simulink model "Standing_Strategy"  (R2025a)
settings: Solver=ode23t  StartTime=0.0  StopTime=4.0  MaxStep=0.01  RelTol=1e-3
InitFcn:
  | params;
values from neighbouring files (symbols this model uses):
  ankle = []    [params.m]
  arm = []    [params.m]
  F_inp = 70    [params.m]
  foot = []    [params.m]
  g = 9.81    [params.m]
  heel = []    [params.m]
  hip_joint = []    [params.m]
  leg = []    [params.m]
  mp = []    [params.m]
  shoulder = []    [params.m]
  sol = []    [params.m]
  ta = []    [params.m]
  torso = []    [params.m]
undefined symbols (not defined in the file or in its folder): X, Y, Z
libraries: sm_lib x43, nesl_utility x13, dlactivationlib x2
(part 2 of 2)

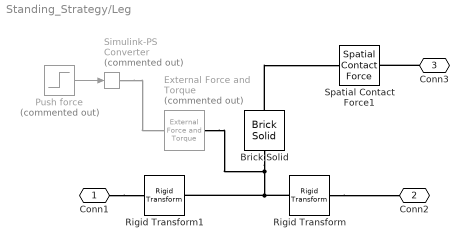
== system Standing_Strategy/Leg ==
  Brick Solid : sm_lib/Body Elements/Brick Solid  BrickDimensions=[L W H]  BrickDimensionsUnits=m  ExportEntireGeometry=on  InertiaType=CalculateFromGeometry  BasedOnType=Density  Density=rho  DensityUnits=g/cm^3  Mass=1  MassUnits=kg  CenterOfMass=[0 0 0]  CenterOfMassUnits=m  MomentsOfInertia=[1 1 1]  MomentsOfInertiaUnits=kg*m^2  ProductsOfInertia=[0 0 0]  ProductsOfInertiaUnits=kg*m^2  GraphicType=FromGeometry  MarkerShape=Sphere  MarkerSize=10  GraphicVisPropType=SimpleVisualProperties  GraphicDiffuseColor=rgb  GraphicOpacity=1  GraphicSpecularColor=[0.5 0.5 0.5 1.0]  GraphicAmbientColor=[0.15 0.15 0.15 1.0]  GraphicEmissiveColor=[0.0 0.0 0.0 1.0]  GraphicShininess=75  DoExposeReferenceFrame=on  SerializedFrames=<Frames/>
  External Force and Torque : sm_lib/Forces and Torques/External Force and Torque  Commented=on  EnableForceX=off  EnableForceY=off  EnableForceZ=on  EnableForce=off  ForceResolutionFrame=AttachedFrame  EnableTorqueX=off  EnableTorqueY=off  EnableTorqueZ=off  EnableTorque=off  TorqueResolutionFrame=AttachedFrame
  Push force : Step  Commented=on  Time=0.1  Before=-300  After=0  SampleTime=0
  Rigid Transform : sm_lib/Frames and Transforms/Rigid Transform  RotationMethod=None  FollAlignAxisA=+X  BaseAlignAxisA=+Y  FollAlignAxisB=+Y  BaseAlignAxisB=+Z  RotationStandardAxis=+Y  RotationAngle=-90  RotationAngleUnits=deg  RotationArbitraryAxis=[0 0 1]  RotationSequenceAxes=FollowerAxes  RotationSequence=XYX  RotationSequenceAngles=[0 0 0]  RotationSequenceAnglesUnits=deg  RotationMatrix=[1 0 0; 0 1 0; 0 0 1]  Quaternion=[1 0 0 0]  TranslationMethod=StandardAxis  TranslationCartesianOffset=[0 0 0]  TranslationCartesianOffsetUnits=m  TranslationStandardAxis=+X  TranslationStandardOffset=L/2  TranslationStandardOffsetUnits=m  TranslationROffset=0  TranslationROffsetUnits=m  TranslationThetaOffset=0  TranslationThetaOffsetUnits=deg  TranslationZOffset=0  TranslationZOffsetUnits=m
  Rigid Transform1 : sm_lib/Frames and Transforms/Rigid Transform  RotationMethod=None  FollAlignAxisA=+X  BaseAlignAxisA=+Y  FollAlignAxisB=+Y  BaseAlignAxisB=+Z  RotationStandardAxis=+Y  RotationAngle=-90  RotationAngleUnits=deg  RotationArbitraryAxis=[0 0 1]  RotationSequenceAxes=FollowerAxes  RotationSequence=XYX  RotationSequenceAngles=[0 0 0]  RotationSequenceAnglesUnits=deg  RotationMatrix=[1 0 0; 0 1 0; 0 0 1]  Quaternion=[1 0 0 0]  TranslationMethod=StandardAxis  TranslationCartesianOffset=[0 0 0]  TranslationCartesianOffsetUnits=m  TranslationStandardAxis=-X  TranslationStandardOffset=L/2  TranslationStandardOffsetUnits=m  TranslationROffset=0  TranslationROffsetUnits=m  TranslationThetaOffset=0  TranslationThetaOffsetUnits=deg  TranslationZOffset=0  TranslationZOffsetUnits=m
  Simulink-PS Converter : nesl_utility/Simulink-PS Converter  Commented=on  PhysicalDomain=network_engine_domain  SubClassName=ps_input  LeftPortType=input  RightPortType=output  PseudoPeriodic=off  Frequencies=[]  NoiseDistribution=none  NoiseParameters=[]  Unit=1  AffineConversion=off  FilteringAndDerivatives=provide  SimscapeFilterOrder=1  InputFilterTimeConstant=0.001  UdotUserProvided=0
  Spatial Contact Force1 : sm_lib/Forces and Torques/Spatial Contact Force  SenseSeparationDistance=off  NormalForceType=SmoothSpringDamper  NormalStiffness=1e6  NormalStiffnessUnits=N/m  NormalDamping=1e3  NormalDampingUnits=N/(m/s)  NormalTransitionRegionWidth=1e-4  NormalTransitionRegionWidthUnits=m  FrictionType=SmoothStickSlip  CoefficientOfStaticFriction=0.2  CoefficientOfDynamicFriction=0.1  FrictionalCriticalVelocity=1e-3  FrictionalCriticalVelocityUnits=m/s  SenseContactSignal=off  SensePenetrationDepth=off  SenseNormalVelocity=off  SenseTangentialVelocity=off  SensingForceTorqueDirection=BaseOnFollower  SensingForceTorqueResolutionFrame=ContactFrame  SenseNormalForce=off  SenseNormalForceMagnitude=off  SenseNormalTorque=off  SenseFrictionalForce=off  SenseFrictionalForceMagnitude=off  SenseFrictionalTorque=off  SenseTotalForce=off  SenseTotalTorque=off  SenseContactBaseRotation=off  SenseContactBaseTranslation=off  SenseContactFollowerRotation=off  SenseContactFollowerTranslation=off  ZeroCrossDetectContactStartAndEnd=off
  Conn1 : PMIOPort  Side=Left
  Conn2 : PMIOPort  Port=2  Side=Right
  Conn3 : PMIOPort  Port=3  Side=Right
  wires:
  Push force/1 -> Simulink-PS Converter/1
  connections:
  Rigid Transform/RConn1 -- Conn2/RConn1
  Conn1/RConn1 -- Rigid Transform1/RConn1
  Brick Solid/RConn1 -- External Force and Torque/RConn1 -- Rigid Transform/LConn1 -- Rigid Transform1/LConn1
  Brick Solid/LConn1 -- Spatial Contact Force1/RConn1
  Conn3/RConn1 -- Spatial Contact Force1/LConn1
  Simulink-PS Converter/RConn1 -- External Force and Torque/LConn1

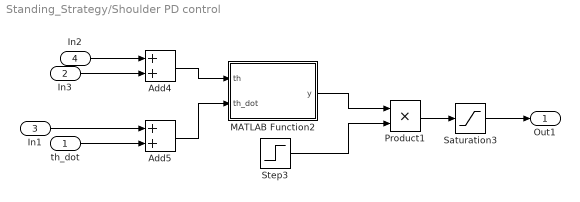
== system Standing_Strategy/Shoulder PD control ==
  th_dot : Inport
  In3 : Inport  Port=2
  In1 : Inport  Port=3
  In2 : Inport  Port=4
  Add4 : Sum
  Add5 : Sum
  MATLAB Function2 : MATLAB Function  TreatAsAtomicUnit=on
  Product1 : Product
  Saturation3 : Saturate  UpperLimit=50  LowerLimit=-50
  Step3 : Step  Time=10*hip_joint.T2  SampleTime=0
  Out1 : Outport
  wires:
  Product1/1 -> Saturation3/1
  Add5/1 -> MATLAB Function2/2(th_dot)
  In1/1 -> Add5/1
  Step3/1 -> Product1/2
  Add4/1 -> MATLAB Function2/1(th)
  In2/1 -> Add4/1
  MATLAB Function2/1(y) -> Product1/1
  In3/1 -> Add4/2
  th_dot/1 -> Add5/2
  Saturation3/1 -> Out1/1

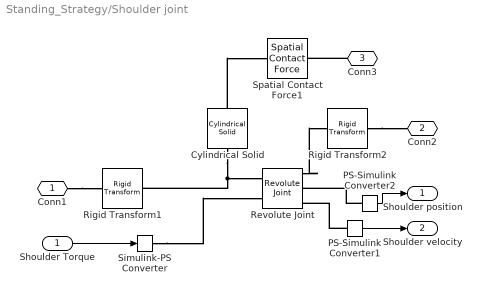
== system Standing_Strategy/Shoulder joint ==
  Shoulder Torque : Inport
  Cylindrical Solid : sm_lib/Body Elements/Cylindrical Solid  CylinderRadius=R  CylinderRadiusUnits=m  CylinderLength=L  CylinderLengthUnits=m  ExportEntireGeometry=on  InertiaType=CalculateFromGeometry  BasedOnType=Density  Density=rho  DensityUnits=g/cm^3  Mass=1  MassUnits=kg  CenterOfMass=[0 0 0]  CenterOfMassUnits=m  MomentsOfInertia=[1 1 1]  MomentsOfInertiaUnits=kg*m^2  ProductsOfInertia=[0 0 0]  ProductsOfInertiaUnits=kg*m^2  GraphicType=FromGeometry  MarkerShape=Sphere  MarkerSize=10  GraphicVisPropType=SimpleVisualProperties  GraphicDiffuseColor=rgb  GraphicOpacity=1  GraphicSpecularColor=[0.5 0.5 0.5 1.0]  GraphicAmbientColor=[0.15 0.15 0.15 1.0]  GraphicEmissiveColor=[0.0 0.0 0.0 1.0]  GraphicShininess=75  DoExposeReferenceFrame=on  SerializedFrames=<Frames/>
  PS-Simulink Converter1 : nesl_utility/PS-Simulink Converter  PhysicalDomain=network_engine_domain  SubClassName=ps_output  LeftPortType=input  RightPortType=output  PseudoPeriodic=off  Frequencies=[]  VectorFormat=inherit  Unit=inherit  AffineConversion=off
  PS-Simulink Converter2 : nesl_utility/PS-Simulink Converter  PhysicalDomain=network_engine_domain  SubClassName=ps_output  LeftPortType=input  RightPortType=output  PseudoPeriodic=off  Frequencies=[]  VectorFormat=inherit  Unit=inherit  AffineConversion=off
  Revolute Joint : sm_lib/Joints/Revolute Joint  JointMode=Normal  CompositeWrenchDir=FollowerOnBase  CompositeWrenchFrame=BaseFrame  SenseConstraintForce=off  SenseConstraintTorque=off  SenseTotalForce=off  SenseTotalTorque=off  PositionTargetSpecify=on  PositionTargetPriority=High  PositionTargetValue=shoulder.th_init  PositionTargetValueUnits=rad  VelocityTargetSpecify=off  VelocityTargetPriority=High  VelocityTargetValue=0  VelocityTargetValueUnits=deg/s  EquilibriumPosition=shoulder.th_init  EquilibriumPositionUnits=rad  SpringStiffness=0  SpringStiffnessUnits=N*m/deg  DampingCoefficient=0.1  DampingCoefficientUnits=N*m/(deg/s)  LowerLimitSpecify=off  LowerLimitBound=0  LowerLimitBoundUnits=deg  LowerLimitStiffness=1e4  LowerLimitStiffnessUnits=N*m/deg  LowerLimitDamping=10  LowerLimitDampingUnits=N*m/(deg/s)  LowerLimitTransitionRegionWidth=0.1  LowerLimitTransitionRegionWidthUnits=deg  UpperLimitSpecify=off  UpperLimitBound=120  UpperLimitBoundUnits=deg  UpperLimitStiffness=1e4  UpperLimitStiffnessUnits=N*m/deg  UpperLimitDamping=10  UpperLimitDampingUnits=N*m/(deg/s)  UpperLimitTransitionRegionWidth=0.1  UpperLimitTransitionRegionWidthUnits=deg  TorqueActuationMode=InputTorque  MotionActuationMode=ComputedMotion  SensePosition=on  SenseVelocity=on  SenseAcceleration=off  SenseTorqueForce=off  SenseLowerLimitTorqueForce=off  SenseUpperLimitTorqueForce=off
  Rigid Transform1 : sm_lib/Frames and Transforms/Rigid Transform  RotationMethod=StandardAxis  FollAlignAxisA=+X  BaseAlignAxisA=+Y  FollAlignAxisB=+Y  BaseAlignAxisB=+Z  RotationStandardAxis=+X  RotationAngle=90  RotationAngleUnits=deg  RotationArbitraryAxis=[0 0 1]  RotationSequenceAxes=FollowerAxes  RotationSequence=XYX  RotationSequenceAngles=[0 0 0]  RotationSequenceAnglesUnits=deg  RotationMatrix=[1 0 0; 0 1 0; 0 0 1]  Quaternion=[1 0 0 0]  TranslationMethod=StandardAxis  TranslationCartesianOffset=[0 0 0]  TranslationCartesianOffsetUnits=m  TranslationStandardAxis=-X  TranslationStandardOffset=R  TranslationStandardOffsetUnits=m  TranslationROffset=0  TranslationROffsetUnits=m  TranslationThetaOffset=0  TranslationThetaOffsetUnits=deg  TranslationZOffset=0  TranslationZOffsetUnits=m
  Rigid Transform2 : sm_lib/Frames and Transforms/Rigid Transform  RotationMethod=StandardAxis  FollAlignAxisA=+X  BaseAlignAxisA=+Y  FollAlignAxisB=+Y  BaseAlignAxisB=+Z  RotationStandardAxis=-X  RotationAngle=90  RotationAngleUnits=deg  RotationArbitraryAxis=[0 0 1]  RotationSequenceAxes=FollowerAxes  RotationSequence=XYX  RotationSequenceAngles=[0 0 0]  RotationSequenceAnglesUnits=deg  RotationMatrix=[1 0 0; 0 1 0; 0 0 1]  Quaternion=[1 0 0 0]  TranslationMethod=StandardAxis  TranslationCartesianOffset=[0 0 0]  TranslationCartesianOffsetUnits=m  TranslationStandardAxis=-X  TranslationStandardOffset=R  TranslationStandardOffsetUnits=m  TranslationROffset=0  TranslationROffsetUnits=m  TranslationThetaOffset=0  TranslationThetaOffsetUnits=deg  TranslationZOffset=0  TranslationZOffsetUnits=m
  Simulink-PS Converter : nesl_utility/Simulink-PS Converter  PhysicalDomain=network_engine_domain  SubClassName=ps_input  LeftPortType=input  RightPortType=output  PseudoPeriodic=off  Frequencies=[]  NoiseDistribution=none  NoiseParameters=[]  Unit=1  AffineConversion=off  FilteringAndDerivatives=provide  SimscapeFilterOrder=1  InputFilterTimeConstant=0.001  UdotUserProvided=0
  Spatial Contact Force1 : sm_lib/Forces and Torques/Spatial Contact Force  SenseSeparationDistance=off  NormalForceType=SmoothSpringDamper  NormalStiffness=1e6  NormalStiffnessUnits=N/m  NormalDamping=1e3  NormalDampingUnits=N/(m/s)  NormalTransitionRegionWidth=1e-4  NormalTransitionRegionWidthUnits=m  FrictionType=SmoothStickSlip  CoefficientOfStaticFriction=0.2  CoefficientOfDynamicFriction=0.1  FrictionalCriticalVelocity=1e-3  FrictionalCriticalVelocityUnits=m/s  SenseContactSignal=off  SensePenetrationDepth=off  SenseNormalVelocity=off  SenseTangentialVelocity=off  SensingForceTorqueDirection=BaseOnFollower  SensingForceTorqueResolutionFrame=ContactFrame  SenseNormalForce=off  SenseNormalForceMagnitude=off  SenseNormalTorque=off  SenseFrictionalForce=off  SenseFrictionalForceMagnitude=off  SenseFrictionalTorque=off  SenseTotalForce=off  SenseTotalTorque=off  SenseContactBaseRotation=off  SenseContactBaseTranslation=off  SenseContactFollowerRotation=off  SenseContactFollowerTranslation=off  ZeroCrossDetectContactStartAndEnd=off
  Conn1 : PMIOPort  Side=Left
  Conn2 : PMIOPort  Port=2  Side=Right
  Conn3 : PMIOPort  Port=3  Side=Right
  Shoulder position : Outport
  Shoulder velocity : Outport  Port=2
  wires:
  PS-Simulink Converter1/1 -> Shoulder velocity/1
  Shoulder Torque/1 -> Simulink-PS Converter/1
  PS-Simulink Converter2/1 -> Shoulder position/1
  connections:
  Conn1/RConn1 -- Rigid Transform1/RConn1
  Cylindrical Solid/RConn1 -- Rigid Transform1/LConn1 -- Revolute Joint/LConn1
  Cylindrical Solid/LConn1 -- Spatial Contact Force1/RConn1
  Conn3/RConn1 -- Spatial Contact Force1/LConn1
  Rigid Transform2/LConn1 -- Conn2/RConn1
  Revolute Joint/RConn1 -- Rigid Transform2/RConn1
  PS-Simulink Converter1/LConn1 -- Revolute Joint/RConn3
  Simulink-PS Converter/RConn1 -- Revolute Joint/LConn2
  PS-Simulink Converter2/LConn1 -- Revolute Joint/RConn2

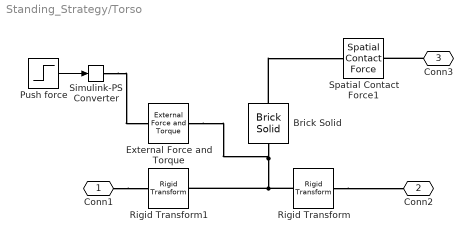
== system Standing_Strategy/Torso ==
  Brick Solid : sm_lib/Body Elements/Brick Solid  BrickDimensions=[L W H]  BrickDimensionsUnits=m  ExportEntireGeometry=on  InertiaType=CalculateFromGeometry  BasedOnType=Density  Density=rho  DensityUnits=g/cm^3  Mass=1  MassUnits=kg  CenterOfMass=[0 0 0]  CenterOfMassUnits=m  MomentsOfInertia=[1 1 1]  MomentsOfInertiaUnits=kg*m^2  ProductsOfInertia=[0 0 0]  ProductsOfInertiaUnits=kg*m^2  GraphicType=FromGeometry  MarkerShape=Sphere  MarkerSize=10  GraphicVisPropType=SimpleVisualProperties  GraphicDiffuseColor=rgb  GraphicOpacity=1  GraphicSpecularColor=[0.5 0.5 0.5 1.0]  GraphicAmbientColor=[0.15 0.15 0.15 1.0]  GraphicEmissiveColor=[0.0 0.0 0.0 1.0]  GraphicShininess=75  DoExposeReferenceFrame=on  SerializedFrames=<Frames/>
  External Force and Torque : sm_lib/Forces and Torques/External Force and Torque  EnableForceX=off  EnableForceY=off  EnableForceZ=on  EnableForce=off  ForceResolutionFrame=AttachedFrame  EnableTorqueX=off  EnableTorqueY=off  EnableTorqueZ=off  EnableTorque=off  TorqueResolutionFrame=AttachedFrame
  Push force : Step  Time=0.1  Before=-F_inp  After=0  SampleTime=0
  Rigid Transform : sm_lib/Frames and Transforms/Rigid Transform  RotationMethod=None  FollAlignAxisA=+X  BaseAlignAxisA=+Y  FollAlignAxisB=+Y  BaseAlignAxisB=+Z  RotationStandardAxis=+Y  RotationAngle=-90  RotationAngleUnits=deg  RotationArbitraryAxis=[0 0 1]  RotationSequenceAxes=FollowerAxes  RotationSequence=XYX  RotationSequenceAngles=[0 0 0]  RotationSequenceAnglesUnits=deg  RotationMatrix=[1 0 0; 0 1 0; 0 0 1]  Quaternion=[1 0 0 0]  TranslationMethod=StandardAxis  TranslationCartesianOffset=[0 0 0]  TranslationCartesianOffsetUnits=m  TranslationStandardAxis=+X  TranslationStandardOffset=L/2  TranslationStandardOffsetUnits=m  TranslationROffset=0  TranslationROffsetUnits=m  TranslationThetaOffset=0  TranslationThetaOffsetUnits=deg  TranslationZOffset=0  TranslationZOffsetUnits=m
  Rigid Transform1 : sm_lib/Frames and Transforms/Rigid Transform  RotationMethod=None  FollAlignAxisA=+X  BaseAlignAxisA=+Y  FollAlignAxisB=+Y  BaseAlignAxisB=+Z  RotationStandardAxis=+Y  RotationAngle=-90  RotationAngleUnits=deg  RotationArbitraryAxis=[0 0 1]  RotationSequenceAxes=FollowerAxes  RotationSequence=XYX  RotationSequenceAngles=[0 0 0]  RotationSequenceAnglesUnits=deg  RotationMatrix=[1 0 0; 0 1 0; 0 0 1]  Quaternion=[1 0 0 0]  TranslationMethod=StandardAxis  TranslationCartesianOffset=[0 0 0]  TranslationCartesianOffsetUnits=m  TranslationStandardAxis=-X  TranslationStandardOffset=L/2  TranslationStandardOffsetUnits=m  TranslationROffset=0  TranslationROffsetUnits=m  TranslationThetaOffset=0  TranslationThetaOffsetUnits=deg  TranslationZOffset=0  TranslationZOffsetUnits=m
  Simulink-PS Converter : nesl_utility/Simulink-PS Converter  PhysicalDomain=network_engine_domain  SubClassName=ps_input  LeftPortType=input  RightPortType=output  PseudoPeriodic=off  Frequencies=[]  NoiseDistribution=none  NoiseParameters=[]  Unit=1  AffineConversion=off  FilteringAndDerivatives=provide  SimscapeFilterOrder=1  InputFilterTimeConstant=0.001  UdotUserProvided=0
  Spatial Contact Force1 : sm_lib/Forces and Torques/Spatial Contact Force  SenseSeparationDistance=off  NormalForceType=SmoothSpringDamper  NormalStiffness=1e6  NormalStiffnessUnits=N/m  NormalDamping=1e3  NormalDampingUnits=N/(m/s)  NormalTransitionRegionWidth=1e-4  NormalTransitionRegionWidthUnits=m  FrictionType=SmoothStickSlip  CoefficientOfStaticFriction=0.2  CoefficientOfDynamicFriction=0.1  FrictionalCriticalVelocity=1e-3  FrictionalCriticalVelocityUnits=m/s  SenseContactSignal=off  SensePenetrationDepth=off  SenseNormalVelocity=off  SenseTangentialVelocity=off  SensingForceTorqueDirection=BaseOnFollower  SensingForceTorqueResolutionFrame=ContactFrame  SenseNormalForce=off  SenseNormalForceMagnitude=off  SenseNormalTorque=off  SenseFrictionalForce=off  SenseFrictionalForceMagnitude=off  SenseFrictionalTorque=off  SenseTotalForce=off  SenseTotalTorque=off  SenseContactBaseRotation=off  SenseContactBaseTranslation=off  SenseContactFollowerRotation=off  SenseContactFollowerTranslation=off  ZeroCrossDetectContactStartAndEnd=off
  Conn1 : PMIOPort  Side=Left
  Conn2 : PMIOPort  Port=2  Side=Right
  Conn3 : PMIOPort  Port=3  Side=Right
  wires:
  Push force/1 -> Simulink-PS Converter/1
  connections:
  Rigid Transform/RConn1 -- Conn2/RConn1
  Conn1/RConn1 -- Rigid Transform1/RConn1
  Brick Solid/RConn1 -- Rigid Transform/LConn1 -- Rigid Transform1/LConn1 -- External Force and Torque/RConn1
  Brick Solid/LConn1 -- Spatial Contact Force1/RConn1
  Conn3/RConn1 -- Spatial Contact Force1/LConn1
  Simulink-PS Converter/RConn1 -- External Force and Torque/LConn1

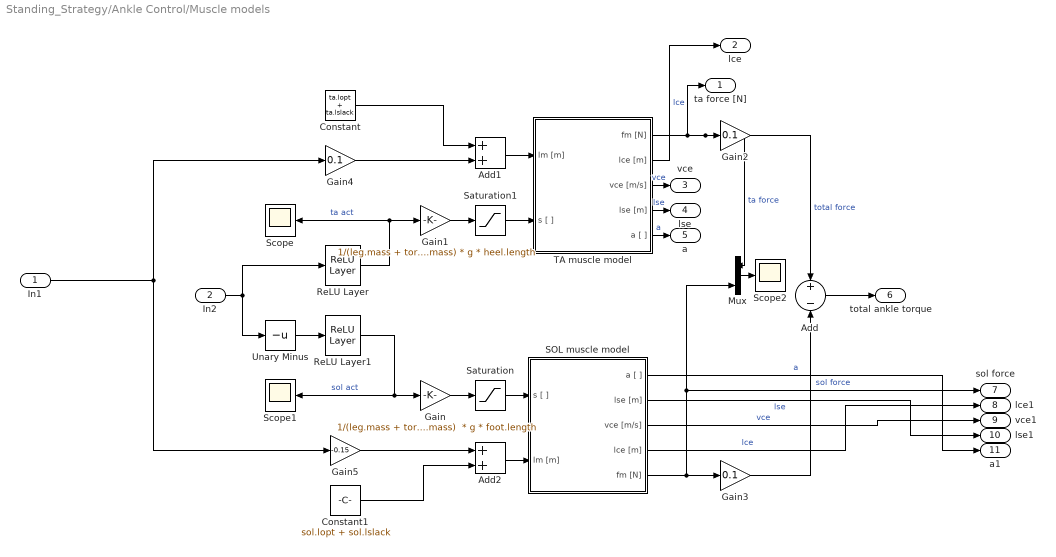
== system Standing_Strategy/Ankle Control/Muscle models ==
  In1 : Inport
  In2 : Inport  Port=2
  Add : Sum  Inputs=+-
  Add1 : Sum
  Add2 : Sum
  Constant : Constant  Value=ta.lopt + ta.lslack
  Constant1 : Constant  Value=sol.lopt + sol.lslack
  Gain : Gain  Gain="1/(leg.mass + torso.mass + arm.mass)  * g * foot.length"
  Gain1 : Gain  Gain=1/(leg.mass + torso.mass + arm.mass) * g * heel.length
  Gain2 : Gain  Gain=0.1
  Gain3 : Gain  Gain=0.1
  Gain4 : Gain  Gain=0.1
  Gain5 : Gain  Gain=-0.15
  Mux : Mux  Inputs=2
  ReLU Layer : dlactivationlib/ReLU Layer  OutMin=[]  OutMax=[]  SampleTime=-1
  ReLU Layer1 : dlactivationlib/ReLU Layer  OutMin=[]  OutMax=[]  SampleTime=-1
  SOL muscle model : Subsystem
  Saturation : Saturate  UpperLimit=1  LowerLimit=0
  Saturation1 : Saturate  UpperLimit=1  LowerLimit=0
  Scope : Scope
      settings: ActiveDisplayYMinimum=-1  ActiveDisplayYMaximum=1  DataLoggingVariableName=ScopeData4
  Scope1 : Scope
      settings: ActiveDisplayYMinimum=-1  ActiveDisplayYMaximum=1  DataLoggingVariableName=ScopeData7
  Scope2 : Scope
      settings: ActiveDisplayYMinimum=-255.71849038678818  ActiveDisplayYMaximum=2301.4664134810942  DataLoggingVariableName=ScopeData8
  TA muscle model : Subsystem
  Unary Minus : UnaryMinus
  ta force [N] : Outport
  lce : Outport  Port=2
  vce : Outport  Port=3
  lse : Outport  Port=4
  a : Outport  Port=5
  total ankle torque : Outport  Port=6
  sol force : Outport  Port=7
  lce1 : Outport  Port=8
  vce1 : Outport  Port=9
  lse1 : Outport  Port=10
  a1 : Outport  Port=11
  wires:
  Mux/1 -> Scope2/1
  Gain3/1 -> Add/2
  Gain2/1 -> Add/1  "total force"
  Add2/1 -> SOL muscle model/2(lm [m])
  TA muscle model/5(a [ ]) -> a/1  "a"
  TA muscle model/1(fm [N]) -> ta force [N]/1, Mux/1, Gain2/1  "ta force"
  Saturation/1 -> SOL muscle model/1(s [ ])
  Constant1/1 -> Add2/2
  Gain5/1 -> Add2/1
  ReLU Layer/1 -> Gain1/1, Scope/1  "ta act"
  SOL muscle model/4(lce [m]) -> lce1/1  "lce"
  In2/1 -> ReLU Layer/1, Unary Minus/1
  SOL muscle model/3(vce [m/s]) -> vce1/1  "vce"
  Add/1 -> total ankle torque/1
  Saturation1/1 -> TA muscle model/2(s [ ])
  Gain1/1 -> Saturation1/1
  SOL muscle model/5(fm [N]) -> sol force/1, Mux/2, Gain3/1  "sol force"
  Gain4/1 -> Add1/2
  ReLU Layer1/1 -> Scope1/1, Gain/1  "sol act"
  In1/1 -> Gain5/1, Gain4/1
  TA muscle model/2(lce [m]) -> lce/1  "lce"
  TA muscle model/4(lse [m]) -> lse/1  "lse"
  SOL muscle model/2(lse [m]) -> lse1/1  "lse"
  Add1/1 -> TA muscle model/1(lm [m])
  TA muscle model/3(vce [m/s]) -> vce/1  "vce"
  Unary Minus/1 -> ReLU Layer1/1
  Constant/1 -> Add1/1
  SOL muscle model/1(a [ ]) -> a1/1  "a"
  Gain/1 -> Saturation/1

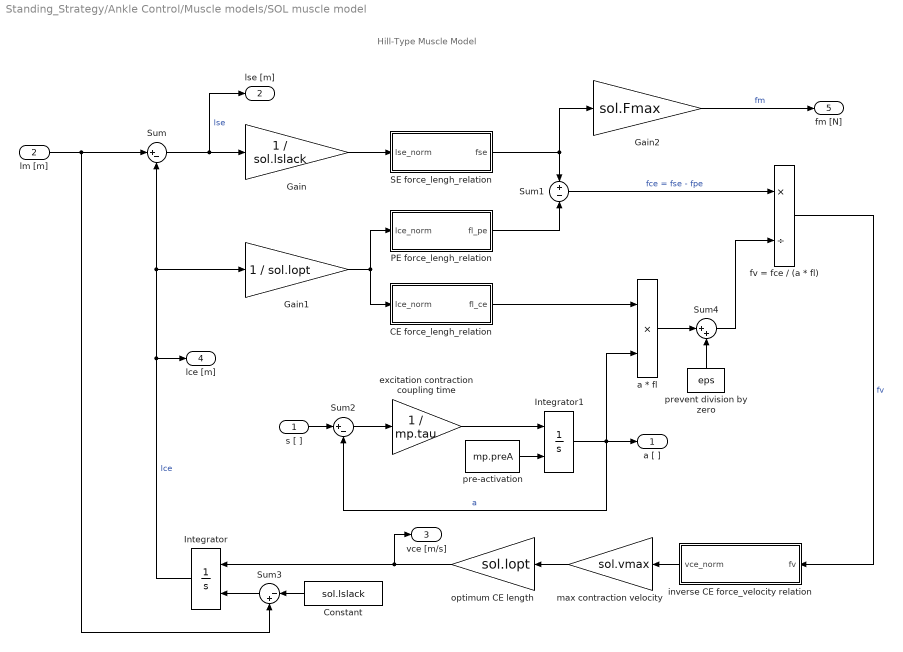
== system Standing_Strategy/Ankle Control/Muscle models/SOL muscle model ==
  note: Hill-Type Muscle Model
  s [ ] : Inport
  lm [m] : Inport  Port=2
  CE force_lengh_relation : MATLAB Function  TreatAsAtomicUnit=on
  Constant : Constant  Value=sol.lslack
  Gain : Gain  Gain=1 / sol.lslack
  Gain1 : Gain  Gain=1 / sol.lopt
  Gain2 : Gain  Gain=sol.Fmax
  Integrator : Integrator  InitialConditionSource=external
  Integrator1 : Integrator  InitialConditionSource=external
  PE force_lengh_relation : MATLAB Function  TreatAsAtomicUnit=on
  SE force_lengh_relation : MATLAB Function  TreatAsAtomicUnit=on
  Sum : Sum  Inputs=|+-
  Sum1 : Sum  Inputs=+-
  Sum2 : Sum  Inputs=|+-
  Sum3 : Sum  Inputs=|-+
  Sum4 : Sum  Inputs=|++
  a * fl : Product  Inputs=**
  excitation contraction coupling time : Gain  Gain=1 / mp.tau
  fv = fce / (a * fl) : Product  Inputs=*/
  inverse CE force_velocity relation : MATLAB Function  TreatAsAtomicUnit=on
  max contraction velocity : Gain  Gain=sol.vmax
  optimum CE length : Gain  Gain=sol.lopt
  pre-activation : Constant  Value=mp.preA
  prevent division by zero : Constant  Value=eps
  a [ ] : Outport
  lse [m] : Outport  Port=2
  vce [m/s] : Outport  Port=3
  lce [m] : Outport  Port=4
  fm [N] : Outport  Port=5
  wires:
  Gain2/1 -> fm [N]/1  "fm"
  optimum CE length/1 -> vce [m/s]/1, Integrator/1
  a * fl/1 -> Sum4/1
  Sum2/1 -> excitation contraction coupling time/1
  Gain/1 -> SE force_lengh_relation/1(lse_norm)
  s [ ]/1 -> Sum2/1
  fv = fce / (a * fl)/1 -> inverse CE force_velocity relation/1(fv)  "fv"
  inverse CE force_velocity relation/1(vce_norm) -> max contraction velocity/1
  Sum/1 -> lse [m]/1, Gain/1  "lse"
  Integrator/1 -> lce [m]/1, Gain1/1, Sum/2  "lce"
  SE force_lengh_relation/1(fse) -> Gain2/1, Sum1/1
  PE force_lengh_relation/1(fl_pe) -> Sum1/2
  max contraction velocity/1 -> optimum CE length/1
  Sum3/1 -> Integrator/2
  pre-activation/1 -> Integrator1/2
  CE force_lengh_relation/1(fl_ce) -> a * fl/1
  lm [m]/1 -> Sum3/2, Sum/1
  Sum4/1 -> fv = fce / (a * fl)/2
  Constant/1 -> Sum3/1
  prevent division by zero/1 -> Sum4/2
  excitation contraction coupling time/1 -> Integrator1/1
  Gain1/1 -> CE force_lengh_relation/1(lce_norm), PE force_lengh_relation/1(lce_norm)
  Integrator1/1 -> a * fl/2, a [ ]/1, Sum2/2  "a"
  Sum1/1 -> fv = fce / (a * fl)/1  "fce = fse - fpe"

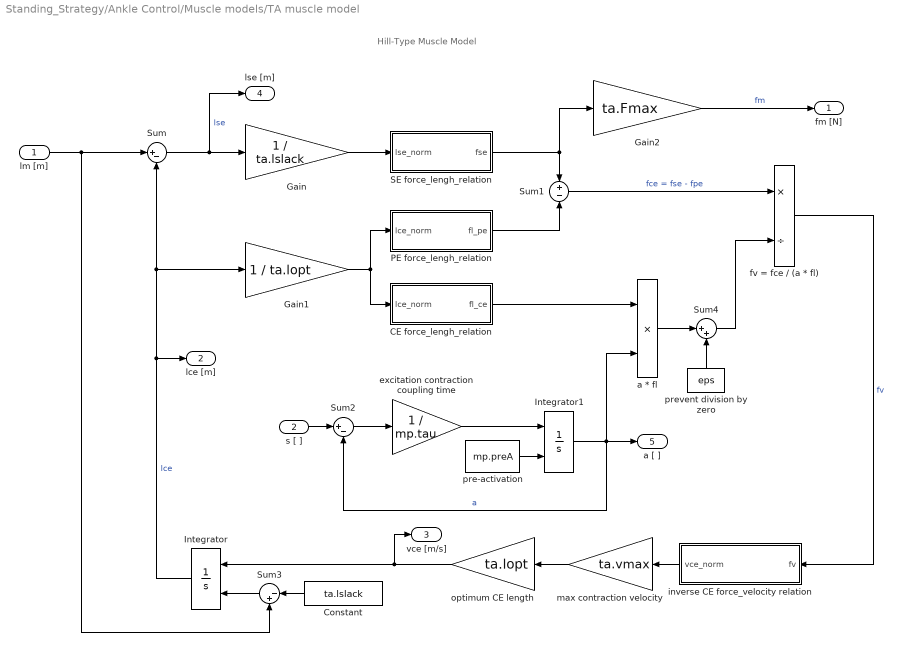
== system Standing_Strategy/Ankle Control/Muscle models/TA muscle model ==
  note: Hill-Type Muscle Model
  lm [m] : Inport
  s [ ] : Inport  Port=2
  CE force_lengh_relation : MATLAB Function  TreatAsAtomicUnit=on
  Constant : Constant  Value=ta.lslack
  Gain : Gain  Gain=1 / ta.lslack
  Gain1 : Gain  Gain=1 / ta.lopt
  Gain2 : Gain  Gain=ta.Fmax
  Integrator : Integrator  InitialConditionSource=external
  Integrator1 : Integrator  InitialConditionSource=external
  PE force_lengh_relation : MATLAB Function  TreatAsAtomicUnit=on
  SE force_lengh_relation : MATLAB Function  TreatAsAtomicUnit=on
  Sum : Sum  Inputs=|+-
  Sum1 : Sum  Inputs=+-
  Sum2 : Sum  Inputs=|+-
  Sum3 : Sum  Inputs=|-+
  Sum4 : Sum  Inputs=|++
  a * fl : Product  Inputs=**
  excitation contraction coupling time : Gain  Gain=1 / mp.tau
  fv = fce / (a * fl) : Product  Inputs=*/
  inverse CE force_velocity relation : MATLAB Function  TreatAsAtomicUnit=on
  max contraction velocity : Gain  Gain=ta.vmax
  optimum CE length : Gain  Gain=ta.lopt
  pre-activation : Constant  Value=mp.preA
  prevent division by zero : Constant  Value=eps
  fm [N] : Outport
  lce [m] : Outport  Port=2
  vce [m/s] : Outport  Port=3
  lse [m] : Outport  Port=4
  a [ ] : Outport  Port=5
  wires:
  Gain2/1 -> fm [N]/1  "fm"
  optimum CE length/1 -> vce [m/s]/1, Integrator/1
  a * fl/1 -> Sum4/1
  Sum2/1 -> excitation contraction coupling time/1
  Gain/1 -> SE force_lengh_relation/1(lse_norm)
  s [ ]/1 -> Sum2/1
  fv = fce / (a * fl)/1 -> inverse CE force_velocity relation/1(fv)  "fv"
  inverse CE force_velocity relation/1(vce_norm) -> max contraction velocity/1
  Sum/1 -> lse [m]/1, Gain/1  "lse"
  Integrator/1 -> lce [m]/1, Gain1/1, Sum/2  "lce"
  SE force_lengh_relation/1(fse) -> Gain2/1, Sum1/1
  PE force_lengh_relation/1(fl_pe) -> Sum1/2
  max contraction velocity/1 -> optimum CE length/1
  Sum3/1 -> Integrator/2
  pre-activation/1 -> Integrator1/2
  CE force_lengh_relation/1(fl_ce) -> a * fl/1
  lm [m]/1 -> Sum3/2, Sum/1
  Sum4/1 -> fv = fce / (a * fl)/2
  Constant/1 -> Sum3/1
  prevent division by zero/1 -> Sum4/2
  excitation contraction coupling time/1 -> Integrator1/1
  Gain1/1 -> CE force_lengh_relation/1(lce_norm), PE force_lengh_relation/1(lce_norm)
  Integrator1/1 -> a * fl/2, a [ ]/1, Sum2/2  "a"
  Sum1/1 -> fv = fce / (a * fl)/1  "fce = fse - fpe"

== matlab function Standing_Strategy/Hip joint PD control/MATLAB Function1 ==
  data: th input; y output; th_dot input; ankle parameter; hip_joint parameter
function y = fcn(th, th_dot, ankle, hip_joint)

    y = hip_joint.kp * ((ankle.th_des + hip_joint.th_des) - th) - hip_joint.kd * th_dot;
end

== matlab function Standing_Strategy/Shoulder PD control/MATLAB Function2 ==
  data: th input; y output; th_dot input; shoulder parameter; ankle parameter; hip_joint parameter
function y = fcn(th, th_dot, shoulder, ankle, hip_joint)

    y = shoulder.kp * (shoulder.th_des + hip_joint.th_des + ankle.th_des - th) - shoulder.kd * th_dot;
end

== matlab function Standing_Strategy/Ankle Control/Muscle models/TA muscle model/CE force_lengh_relation ==
  data: lce_norm input; fl_ce output; mp parameter
function fl_ce = fcn(lce_norm, mp)
% wraps force length relation of contractile element

fl_ce = CE_force_length_relation(lce_norm, mp);

== matlab function Standing_Strategy/Ankle Control/Muscle models/TA muscle model/PE force_lengh_relation ==
  data: lce_norm input; fl_pe output; mp parameter
function fl_pe = fcn(lce_norm, mp)
% wraps force length relation of parallel elasticity

fl_pe = PE_force_length_relation(lce_norm, mp);

== matlab function Standing_Strategy/Ankle Control/Ankle control ==
  data: th input; y output; th_dot input; ankle parameter
function y = fcn(th, th_dot, ankle)

    y = ankle.kp * (ankle.th_des - th) - ankle.kd * th_dot;
end

== matlab function Standing_Strategy/Ankle Control/Muscle models/TA muscle model/SE force_lengh_relation ==
  data: lse_norm input; fse output; mp parameter
function fse = fcn(lse_norm, mp)
% wraps force length relation of series elasticity

fse = SE_force_length_relation(lse_norm, mp);

== matlab function Standing_Strategy/Ankle Control/Muscle models/TA muscle model/inverse CE force_velocity relation ==
  data: fv input; vce_norm output; mp parameter
function vce_norm = fcn(fv, mp)
% wraps inverse force velocity relation of contractile element

vce_norm = CE_inverse_force_velocity_relation(fv, mp);

== matlab function Standing_Strategy/Ankle Control/Muscle models/SOL muscle model/CE force_lengh_relation ==
  data: lce_norm input; fl_ce output; mp parameter
function fl_ce = fcn(lce_norm, mp)
% wraps force length relation of contractile element

fl_ce = CE_force_length_relation(lce_norm, mp);

== matlab function Standing_Strategy/Ankle Control/Muscle models/SOL muscle model/PE force_lengh_relation ==
  data: lce_norm input; fl_pe output; mp parameter
function fl_pe = fcn(lce_norm, mp)
% wraps force length relation of parallel elasticity

fl_pe = PE_force_length_relation(lce_norm, mp);

== matlab function Standing_Strategy/Ankle Control/Muscle models/SOL muscle model/SE force_lengh_relation ==
  data: lse_norm input; fse output; mp parameter
function fse = fcn(lse_norm, mp)
% wraps force length relation of series elasticity

fse = SE_force_length_relation(lse_norm, mp);

== matlab function Standing_Strategy/Ankle Control/Muscle models/SOL muscle model/inverse CE force_velocity relation ==
  data: fv input; vce_norm output; mp parameter
function vce_norm = fcn(fv, mp)
% wraps inverse force velocity relation of contractile element

vce_norm = CE_inverse_force_velocity_relation(fv, mp);
